simulink model "sensors_simulation"  (R2024a)
settings: Solver=VariableStepAuto  StartTime=0.0  StopTime=35  RelTol=1e-3
values from neighbouring files (symbols this model uses):
  t_measure_ms = 1 + 2.3*OSR_T + 2.3*OSR_P + 0.575    (= 42.975)    [main_simu.m]
libraries: aerolibatmos2 x1, dspnetwork x1
settings Model: Creator=andre  LastModifiedBy=andre

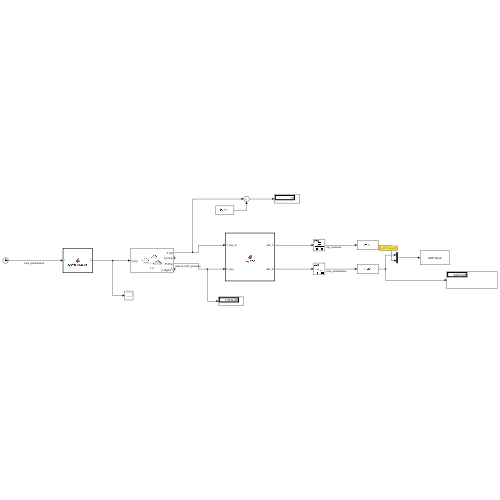
[thumbnail: Simulink's stored preview of the top-level diagram]
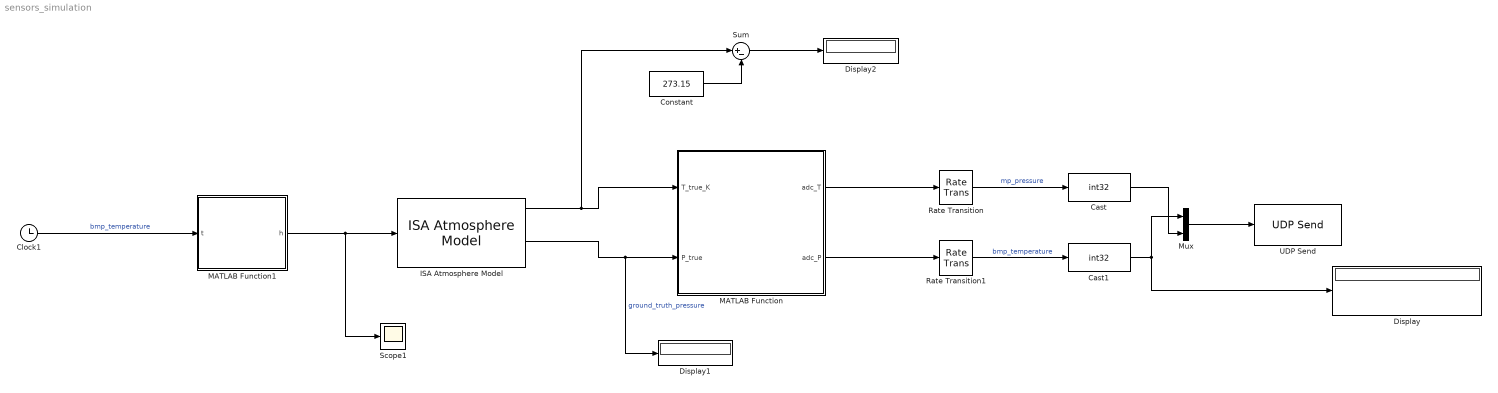
== system sensors_simulation ==
  Cast : DataTypeConversion  OutDataTypeStr=int32  SaturateOnIntegerOverflow=off  RndMeth=Floor
  Cast1 : DataTypeConversion  OutDataTypeStr=int32  SaturateOnIntegerOverflow=off  RndMeth=Floor
  Clock1 : Clock
  Constant : Constant  Value=273.15
  Display : Display
  Display1 : Display
  Display2 : Display
  ISA Atmosphere Model : aerolibatmos2/ISA Atmosphere Model  useExtended=off  action=Warning  custom=off  viscosityOut=off  g=9.80665  gamma=1.4  R=287.0531  L=0.0065  h_trop=11000  h_strat=20000  rho0=1.225  P0=101325  T0=288.15  h0=0  S=110.4  Tref=273.15  muref=1.716e-5
  MATLAB Function : MATLAB Function  TreatAsAtomicUnit=on
  MATLAB Function1 : MATLAB Function  TreatAsAtomicUnit=on
  Mux : Mux  Inputs=2
  Rate Transition : RateTransition  OutPortSampleTime=t_measure_ms / 1000
  Rate Transition1 : RateTransition  OutPortSampleTime=t_measure_ms / 1000
  Scope1 : Scope
  Sum : Sum  Inputs=|+-
  UDP Send : dspnetwork/UDP Send  remoteURL='127.0.0.1'  remotePort=5001  localURL='0.0.0.0'  localPortSource=Automatically determine  localPort=-1  sendBufferSize=8192  sampletime=-1  blockPlatform=[]  separateLengthPort=0
      settings: LibrarySourceBlock=dspsnks4/UDP Send
  wires:
  MATLAB Function/1(adc_T) -> Rate Transition/1
  ISA Atmosphere Model/1 -> Sum/1, MATLAB Function/1(T_true_K)
  MATLAB Function1/1(h) -> Scope1/1, ISA Atmosphere Model/1
  ISA Atmosphere Model/3 -> Display1/1, MATLAB Function/2(P_true)  "ground_truth_pressure"
  MATLAB Function/2(adc_P) -> Rate Transition1/1
  Rate Transition/1 -> Cast/1  "mp_pressure"
  Rate Transition1/1 -> Cast1/1  "bmp_temperature"
  Cast1/1 -> Display/1, Mux/1
  Mux/1 -> UDP Send/1
  Constant/1 -> Sum/2
  Sum/1 -> Display2/1
  Cast/1 -> Mux/2
  Clock1/1 -> MATLAB Function1/1(t)  "bmp_temperature"

== matlab function sensors_simulation/MATLAB Function1 ==
  data: t input; h output
function h = rocket_altitude(t)
% Rocket ascent with delayed ignition
% Phase 0: pre-launch  (0 to t_ign)           — on the pad
% Phase 1: powered     (t_ign to t_ign + t_b)  — constant acceleration
% Phase 2: coast       (after burnout)          — decelerating under gravity

t_ign = 10.0;  % ignition time (seconds)
a     = 30.0;  % m/s² net acceleration during burn (thrust - gravity)
t_b   =  3;  % burn duration (seconds)

v_b       = a * t_b;          % velocity at burnout
h_b       = 0.5 * a * t_b^2; % altitude at burnout
t_burnout = t_ign + t_b;      % absolute burnout time

if t < t_ign
    % Pre-launch: sitting on the pad
    h = 0;

elseif t <= t_burnout
    % Powered phase
    dt = t - t_ign;
    h  = 0.5 * a * dt^2;

else
    % Coast phase (only gravity, no thrust)
    dt = t - t_burnout;
    h  = h_b + v_b * dt - 0.5 * 9.81 * dt^2;
end

% Clamp to ground (handles landing)
h = max(h, 0);
end

== matlab function sensors_simulation/MATLAB Function ==
  data: T_true_K input; P_true input; adc_T output; adc_P output
function [adc_T, adc_P] = bmp280(T_true_K, P_true)

coder.extrinsic('bmp280_model', 'evalin');
OSR_T     = evalin('base', 'OSR_T');
OSR_P     = evalin('base', 'OSR_P');
IIR_coeff = evalin('base', 'IIR_coeff');

adc_P   = 0;
adc_T = 0;

% Call the full BMP280 model
[adc_P, adc_T] = bmp280_model(P_true, T_true_K, OSR_T, OSR_P, IIR_coeff);

end
